simulink model "punto_22"  (R2015a)
settings: Solver=ode45  StartTime=0.0  StopTime=20  RelTol=1e-3
values from neighbouring files (symbols this model uses):
  a = [-6 -11 -6;1 0 0;0 1 0]    [punto_1.m]    (also in punto_2.m = [0 1 0;0 0 1;-5 -6 0]; punto_3.m = [0 1 0;0 0 1;-1.244 -0.3956 -3.145]; punto_4.m = [0 1;0 0])
  b = [1;0;0]    [punto_1.m]    (also in punto_2.m = [0;0;1]; punto_3.m = [0;0;1.244]; punto_4.m = [0;1])
  c = [0 0 10]    [punto_1.m]    (also in punto_2.m = [1 0 0]; punto_3.m = [1 0 0]; punto_4.m = [1 0])
  d = 0    [punto_1.m]    (also in punto_2.m; punto_3.m; punto_4.m)
  k = place(a,b,p)    [punto_1.m]    (also in punto_2.m = acker(a,b,p); punto_3.m = place(a,b,p1); punto_4.m = place(a,b,prealim))
  Ko = acker(a',c',p)'    [punto_2.m]    (also in punto_3.m = place(Abb',Aab',p)'; punto_4.m = place(Abb',Aab',pobsv)')
settings Model: Creator=Jose Roldan  LastModifiedBy=Jose Roldan

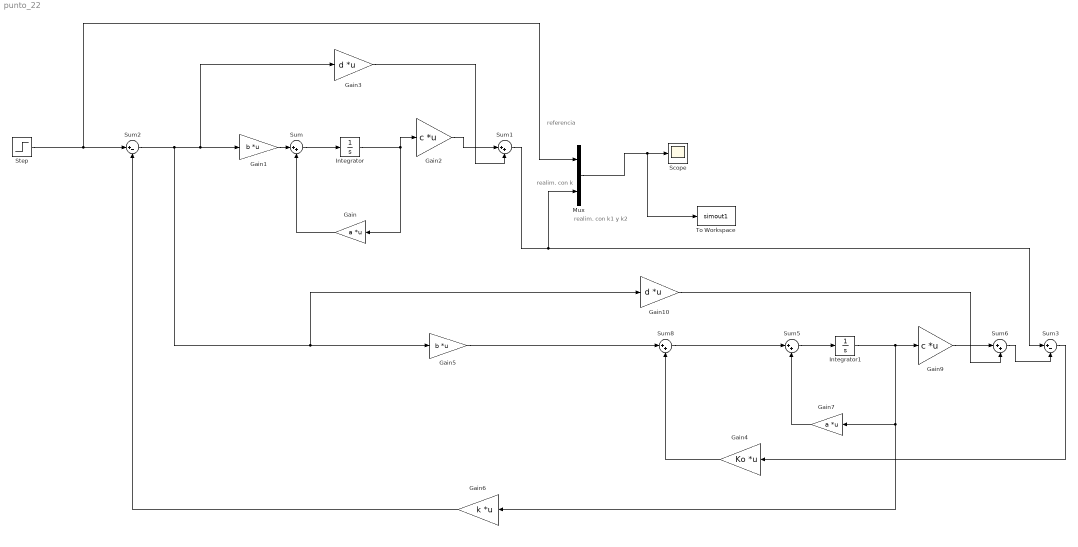
== system punto_22 ==
  note: realim. con k1 y k2
  note: realim. con k
  note: referencia
  Gain : Gain  Gain=a  Multiplication=Matrix(K*u)
  Gain1 : Gain  Gain=b  Multiplication=Matrix(K*u)
  Gain10 : Gain  Gain=d  Multiplication=Matrix(K*u)
  Gain2 : Gain  Gain=c  Multiplication=Matrix(K*u)
  Gain3 : Gain  Gain=d  Multiplication=Matrix(K*u)
  Gain4 : Gain  Gain=Ko  Multiplication=Matrix(K*u)
  Gain5 : Gain  Gain=b  Multiplication=Matrix(K*u)
  Gain6 : Gain  Gain=k  Multiplication=Matrix(K*u)
  Gain7 : Gain  Gain=a  Multiplication=Matrix(K*u)
  Gain9 : Gain  Gain=c  Multiplication=Matrix(K*u)
  Integrator : Integrator
  Integrator1 : Integrator
  Mux : Mux  Inputs=2
  Scope : Scope
  Step : Step  SampleTime=0
  Sum{,1,5..6,8} (5 alike) : Sum  Inputs=|++
  Sum2 : Sum  Inputs=|+-
  Sum3 : Sum  Inputs=|+-
  To Workspace : ToWorkspace  VariableName=simout1  SaveFormat=Timeseries  SampleTime=-1
  wires:
  Step/1 -> Sum2/1, Mux/1
  Gain1/1 -> Sum/1
  Sum/1 -> Integrator/1
  Integrator/1 -> Gain/1, Gain2/1
  Gain2/1 -> Sum1/1
  Gain3/1 -> Sum1/2
  Gain/1 -> Sum/2
  Sum8/1 -> Sum5/1
  Sum5/1 -> Integrator1/1
  Integrator1/1 -> Gain6/1, Gain7/1, Gain9/1
  Gain9/1 -> Sum6/1
  Gain10/1 -> Sum6/2
  Gain7/1 -> Sum5/2
  Sum6/1 -> Sum3/2
  Mux/1 -> To Workspace/1, Scope/1
  Gain5/1 -> Sum8/1
  Gain4/1 -> Sum8/2
  Sum1/1 -> Mux/2, Sum3/1
  Sum3/1 -> Gain4/1
  Sum2/1 -> Gain3/1, Gain1/1, Gain10/1, Gain5/1
  Gain6/1 -> Sum2/2
